simulink model "Demo_TollSystem_cs"  (Simulink 7.6)
settings: Solver=FixedStepDiscrete  SolverMode=SingleTasking  StartTime=0.0  StopTime=13  FixedStep=1/20  RelTol=1e-3
PreLoadFcn:
  | check_NUTS_defined
  | model_closed = 0;
  | assignin('base',['model_closed_' bdroot],false);
InitFcn:
  | PreScanExperimentInitFcn(bdroot)
StopFcn:
  | PreScanExperimentStopFcn(bdroot)
libraries: simulink x9, PreScanUsefulBlocks x6, PreScanSimulinkLibrary x4
(part 2 of 2)

== system Demo_TollSystem_cs/HighwayOverhang_1/RFBeacon_1_Tx_Mux ==
  BeaconType : Inport
  spare_1 : Inport  Port=2
  spare_2 : Inport  Port=3
  spare_3 : Inport  Port=4
  spare_4 : Inport  Port=5
  spare_5 : Inport  Port=6
  spare_6 : Inport  Port=7
  spare_7 : Inport  Port=8
  spare_8 : Inport  Port=9
  spare_9 : Inport  Port=10
  spare_10 : Inport  Port=11
  spare_11 : Inport  Port=12
  spare_12 : Inport  Port=13
  spare_13 : Inport  Port=14
  spare_14 : Inport  Port=15
  spare_15 : Inport  Port=16
  Mux1 : Mux  Inputs=16
  BeaconTx : Outport
  wires:
  BeaconType/1 -> Mux1/1
  spare_11/1 -> Mux1/12
  spare_12/1 -> Mux1/13
  spare_13/1 -> Mux1/14
  spare_14/1 -> Mux1/15
  spare_15/1 -> Mux1/16
  spare_1/1 -> Mux1/2
  spare_2/1 -> Mux1/3
  spare_3/1 -> Mux1/4
  spare_4/1 -> Mux1/5
  spare_5/1 -> Mux1/6
  spare_6/1 -> Mux1/7
  spare_7/1 -> Mux1/8
  spare_8/1 -> Mux1/9
  spare_9/1 -> Mux1/10
  spare_10/1 -> Mux1/11
  Mux1/1 -> BeaconTx/1

== system Demo_TollSystem_cs/HighwayOverhang_1/threshold check ==
  Lat : Inport
  Lon : Inport  Port=2
  Pos Lat : Inport  Port=3
  Pos Lon : Inport  Port=4
  Abs : Abs
  Abs1 : Abs
  Accuracy : Constant  Value=1e-5
  Compare To Zero : simulink/Logic and Bit Operations/Compare To Zero  SystemSampleTime=-1  relop=~=  LogicOutDataTypeMode=uint8  ZeroCross=off
  Compare To Zero1 : simulink/Logic and Bit Operations/Compare To Zero  SystemSampleTime=-1  relop=~=  LogicOutDataTypeMode=uint8  ZeroCross=off
  Logical Operator : Logic  Inputs=3  AllPortsSameDT=off  OutDataTypeStr=boolean
  Logical Operator1 : Logic  Operator=OR  AllPortsSameDT=off  OutDataTypeStr=boolean
  Relational Operator : RelationalOperator  Operator=>  OutDataTypeStr=boolean
  Relational Operator1 : RelationalOperator  Operator=>  OutDataTypeStr=boolean
  Sum : Sum  Inputs=|+-
  Sum1 : Sum  Inputs=|+-
  Out : Outport
  wires:
  Pos Lat/1 -> Sum/2
  Lat/1 -> Sum/1, Compare To Zero/1
  Sum/1 -> Abs/1
  Pos Lon/1 -> Sum1/2
  Lon/1 -> Sum1/1, Compare To Zero1/1
  Sum1/1 -> Abs1/1
  Relational Operator/1 -> Logical Operator1/1
  Logical Operator/1 -> Out/1
  Abs/1 -> Relational Operator/1
  Accuracy/1 -> Relational Operator/2, Relational Operator1/2
  Abs1/1 -> Relational Operator1/1
  Compare To Zero/1 -> Logical Operator/1
  Compare To Zero1/1 -> Logical Operator1/2
  Relational Operator1/1 -> Logical Operator/3
  Logical Operator1/1 -> Logical Operator/2

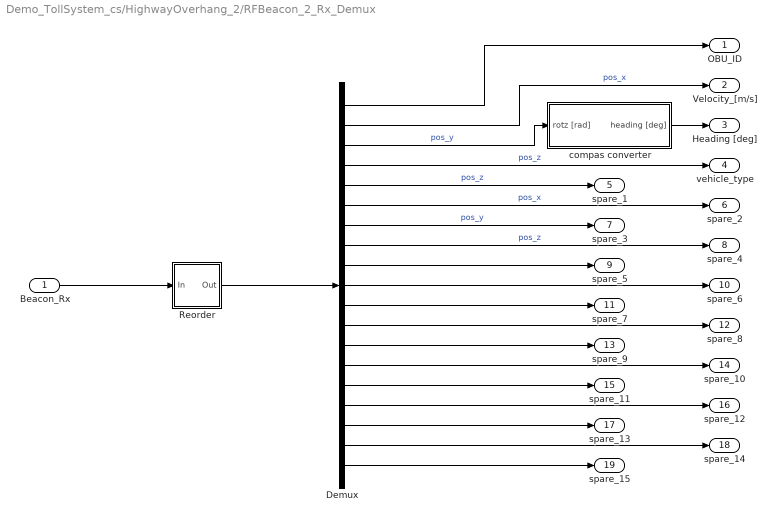
== system Demo_TollSystem_cs/HighwayOverhang_2/RFBeacon_2_Rx_Demux ==
  Beacon_Rx : Inport
  Demux : Demux  Outputs=19
  Reorder : Subsystem  mask(Output reorder block){NrOfOutputs=19, NrOfObjects=5}
      mask prompts: NrOfOutputs "Number Of Outputs [-]"; NrOfObjects "Number Of Objects [-]"
      mask help: Change output order from object based to output type based
      mask init: same as Demo_TollSystem_cs/HighwayOverhang_1/RFBeacon_1_Rx_Demux/Reorder
  compas converter : Subsystem
  OBU_ID : Outport
  Velocity_[m/s] : Outport  Port=2
  Heading [deg] : Outport  Port=3
  vehicle_type : Outport  Port=4
  spare_1 : Outport  Port=5
  spare_2 : Outport  Port=6
  spare_3 : Outport  Port=7
  spare_4 : Outport  Port=8
  spare_5 : Outport  Port=9
  spare_6 : Outport  Port=10
  spare_7 : Outport  Port=11
  spare_8 : Outport  Port=12
  spare_9 : Outport  Port=13
  spare_10 : Outport  Port=14
  spare_11 : Outport  Port=15
  spare_12 : Outport  Port=16
  spare_13 : Outport  Port=17
  spare_14 : Outport  Port=18
  spare_15 : Outport  Port=19
  wires:
  compas converter/1(heading [deg]) -> Heading [deg]/1
  Demux/1 -> OBU_ID/1
  Demux/3 -> compas converter/1(rotz [rad])  "pos_y"
  Demux/2 -> Velocity_[m/s]/1  "pos_x"
  Reorder/1(Out) -> Demux/1
  Demux/5 -> spare_1/1  "pos_z"
  Demux/6 -> spare_2/1  "pos_x"
  Demux/7 -> spare_3/1  "pos_y"
  Demux/8 -> spare_4/1  "pos_z"
  Demux/9 -> spare_5/1
  Demux/10 -> spare_6/1
  Demux/11 -> spare_7/1
  Demux/12 -> spare_8/1
  Demux/13 -> spare_9/1
  Demux/14 -> spare_10/1
  Beacon_Rx/1 -> Reorder/1(In)
  Demux/4 -> vehicle_type/1  "pos_z"
  Demux/15 -> spare_11/1
  Demux/16 -> spare_12/1
  Demux/17 -> spare_13/1
  Demux/18 -> spare_14/1
  Demux/19 -> spare_15/1

== system Demo_TollSystem_cs/HighwayOverhang_2/RFBeacon_2_Tx_Mux ==
  BeaconType : Inport
  spare_1 : Inport  Port=2
  spare_2 : Inport  Port=3
  spare_3 : Inport  Port=4
  spare_4 : Inport  Port=5
  spare_5 : Inport  Port=6
  spare_6 : Inport  Port=7
  spare_7 : Inport  Port=8
  spare_8 : Inport  Port=9
  spare_9 : Inport  Port=10
  spare_10 : Inport  Port=11
  spare_11 : Inport  Port=12
  spare_12 : Inport  Port=13
  spare_13 : Inport  Port=14
  spare_14 : Inport  Port=15
  spare_15 : Inport  Port=16
  Mux1 : Mux  Inputs=16
  BeaconTx : Outport
  wires:
  BeaconType/1 -> Mux1/1
  spare_11/1 -> Mux1/12
  spare_12/1 -> Mux1/13
  spare_13/1 -> Mux1/14
  spare_14/1 -> Mux1/15
  spare_15/1 -> Mux1/16
  spare_1/1 -> Mux1/2
  spare_2/1 -> Mux1/3
  spare_3/1 -> Mux1/4
  spare_4/1 -> Mux1/5
  spare_5/1 -> Mux1/6
  spare_6/1 -> Mux1/7
  spare_7/1 -> Mux1/8
  spare_8/1 -> Mux1/9
  spare_9/1 -> Mux1/10
  spare_10/1 -> Mux1/11
  Mux1/1 -> BeaconTx/1

== system Demo_TollSystem_cs/HighwayOverhang_2/threshold check ==
  Lat : Inport
  Lon : Inport  Port=2
  Pos Lat : Inport  Port=3
  Pos Lon : Inport  Port=4
  Abs : Abs
  Abs1 : Abs
  Accuracy : Constant  Value=1e-5
  Compare To Zero : simulink/Logic and Bit Operations/Compare To Zero  SystemSampleTime=-1  relop=~=  LogicOutDataTypeMode=uint8  ZeroCross=off
  Compare To Zero1 : simulink/Logic and Bit Operations/Compare To Zero  SystemSampleTime=-1  relop=~=  LogicOutDataTypeMode=uint8  ZeroCross=off
  Logical Operator : Logic  Inputs=3  AllPortsSameDT=off  OutDataTypeStr=float('double')
  Logical Operator1 : Logic  Operator=OR  AllPortsSameDT=off  OutDataTypeStr=boolean
  Relational Operator : RelationalOperator  Operator=>  OutDataTypeStr=boolean
  Relational Operator1 : RelationalOperator  Operator=>  OutDataTypeStr=boolean
  Sum : Sum  Inputs=|+-
  Sum1 : Sum  Inputs=|+-
  Out : Outport
  wires:
  Pos Lat/1 -> Sum/2
  Lat/1 -> Sum/1, Compare To Zero/1
  Sum/1 -> Abs/1
  Pos Lon/1 -> Sum1/2
  Lon/1 -> Sum1/1, Compare To Zero1/1
  Sum1/1 -> Abs1/1
  Relational Operator/1 -> Logical Operator1/1
  Logical Operator/1 -> Out/1
  Abs/1 -> Relational Operator/1
  Accuracy/1 -> Relational Operator/2, Relational Operator1/2
  Abs1/1 -> Relational Operator1/1
  Compare To Zero/1 -> Logical Operator/1
  Compare To Zero1/1 -> Logical Operator1/2
  Relational Operator1/1 -> Logical Operator/3
  Logical Operator1/1 -> Logical Operator/2

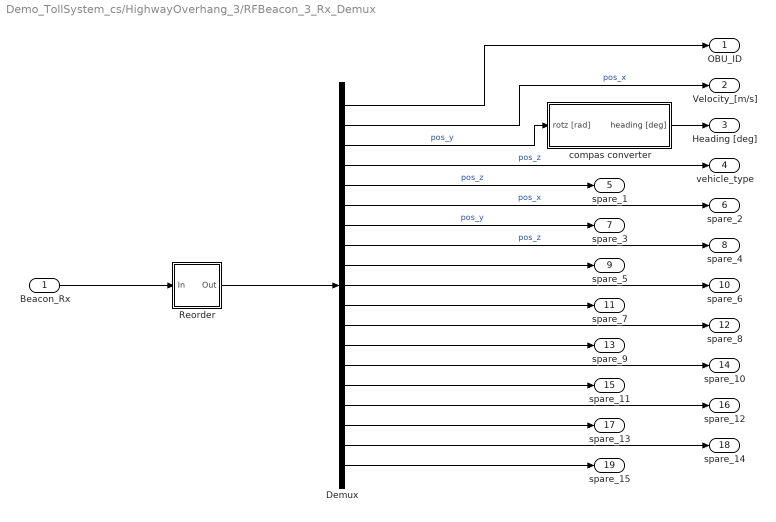
== system Demo_TollSystem_cs/HighwayOverhang_3/RFBeacon_3_Rx_Demux ==
  Beacon_Rx : Inport
  Demux : Demux  Outputs=19
  Reorder : Subsystem  mask(Output reorder block){NrOfOutputs=19, NrOfObjects=5}
      mask prompts: NrOfOutputs "Number Of Outputs [-]"; NrOfObjects "Number Of Objects [-]"
      mask help: Change output order from object based to output type based
      mask init: same as Demo_TollSystem_cs/HighwayOverhang_1/RFBeacon_1_Rx_Demux/Reorder
  compas converter : Subsystem
  OBU_ID : Outport
  Velocity_[m/s] : Outport  Port=2
  Heading [deg] : Outport  Port=3
  vehicle_type : Outport  Port=4
  spare_1 : Outport  Port=5
  spare_2 : Outport  Port=6
  spare_3 : Outport  Port=7
  spare_4 : Outport  Port=8
  spare_5 : Outport  Port=9
  spare_6 : Outport  Port=10
  spare_7 : Outport  Port=11
  spare_8 : Outport  Port=12
  spare_9 : Outport  Port=13
  spare_10 : Outport  Port=14
  spare_11 : Outport  Port=15
  spare_12 : Outport  Port=16
  spare_13 : Outport  Port=17
  spare_14 : Outport  Port=18
  spare_15 : Outport  Port=19
  wires:
  compas converter/1(heading [deg]) -> Heading [deg]/1
  Demux/1 -> OBU_ID/1
  Demux/3 -> compas converter/1(rotz [rad])  "pos_y"
  Demux/2 -> Velocity_[m/s]/1  "pos_x"
  Reorder/1(Out) -> Demux/1
  Demux/5 -> spare_1/1  "pos_z"
  Demux/6 -> spare_2/1  "pos_x"
  Demux/7 -> spare_3/1  "pos_y"
  Demux/8 -> spare_4/1  "pos_z"
  Demux/9 -> spare_5/1
  Demux/10 -> spare_6/1
  Demux/11 -> spare_7/1
  Demux/12 -> spare_8/1
  Demux/13 -> spare_9/1
  Demux/14 -> spare_10/1
  Beacon_Rx/1 -> Reorder/1(In)
  Demux/4 -> vehicle_type/1  "pos_z"
  Demux/15 -> spare_11/1
  Demux/16 -> spare_12/1
  Demux/17 -> spare_13/1
  Demux/18 -> spare_14/1
  Demux/19 -> spare_15/1

== system Demo_TollSystem_cs/HighwayOverhang_3/RFBeacon_3_Tx_Mux ==
  BeaconType : Inport
  spare_1 : Inport  Port=2
  spare_2 : Inport  Port=3
  spare_3 : Inport  Port=4
  spare_4 : Inport  Port=5
  spare_5 : Inport  Port=6
  spare_6 : Inport  Port=7
  spare_7 : Inport  Port=8
  spare_8 : Inport  Port=9
  spare_9 : Inport  Port=10
  spare_10 : Inport  Port=11
  spare_11 : Inport  Port=12
  spare_12 : Inport  Port=13
  spare_13 : Inport  Port=14
  spare_14 : Inport  Port=15
  spare_15 : Inport  Port=16
  Mux1 : Mux  Inputs=16
  BeaconTx : Outport
  wires:
  BeaconType/1 -> Mux1/1
  spare_11/1 -> Mux1/12
  spare_12/1 -> Mux1/13
  spare_13/1 -> Mux1/14
  spare_14/1 -> Mux1/15
  spare_15/1 -> Mux1/16
  spare_1/1 -> Mux1/2
  spare_2/1 -> Mux1/3
  spare_3/1 -> Mux1/4
  spare_4/1 -> Mux1/5
  spare_5/1 -> Mux1/6
  spare_6/1 -> Mux1/7
  spare_7/1 -> Mux1/8
  spare_8/1 -> Mux1/9
  spare_9/1 -> Mux1/10
  spare_10/1 -> Mux1/11
  Mux1/1 -> BeaconTx/1

== system Demo_TollSystem_cs/HighwayOverhang_3/threshold check ==
  Lat : Inport
  Lon : Inport  Port=2
  Pos Lat : Inport  Port=3
  Pos Lon : Inport  Port=4
  Abs : Abs
  Abs1 : Abs
  Accuracy : Constant  Value=1e-5
  Compare To Zero : simulink/Logic and Bit Operations/Compare To Zero  SystemSampleTime=-1  relop=~=  LogicOutDataTypeMode=uint8  ZeroCross=off
  Compare To Zero1 : simulink/Logic and Bit Operations/Compare To Zero  SystemSampleTime=-1  relop=~=  LogicOutDataTypeMode=uint8  ZeroCross=off
  Logical Operator : Logic  Inputs=3  AllPortsSameDT=off  OutDataTypeStr=float('double')
  Logical Operator1 : Logic  Operator=OR  AllPortsSameDT=off  OutDataTypeStr=boolean
  Relational Operator : RelationalOperator  Operator=>  OutDataTypeStr=boolean
  Relational Operator1 : RelationalOperator  Operator=>  OutDataTypeStr=boolean
  Sum : Sum  Inputs=|+-
  Sum1 : Sum  Inputs=|+-
  Out : Outport
  wires:
  Pos Lat/1 -> Sum/2
  Lat/1 -> Sum/1, Compare To Zero/1
  Sum/1 -> Abs/1
  Pos Lon/1 -> Sum1/2
  Lon/1 -> Sum1/1, Compare To Zero1/1
  Sum1/1 -> Abs1/1
  Relational Operator/1 -> Logical Operator1/1
  Logical Operator/1 -> Out/1
  Abs/1 -> Relational Operator/1
  Accuracy/1 -> Relational Operator/2, Relational Operator1/2
  Abs1/1 -> Relational Operator1/1
  Compare To Zero/1 -> Logical Operator/1
  Compare To Zero1/1 -> Logical Operator1/2
  Relational Operator1/1 -> Logical Operator/3
  Logical Operator1/1 -> Logical Operator/2

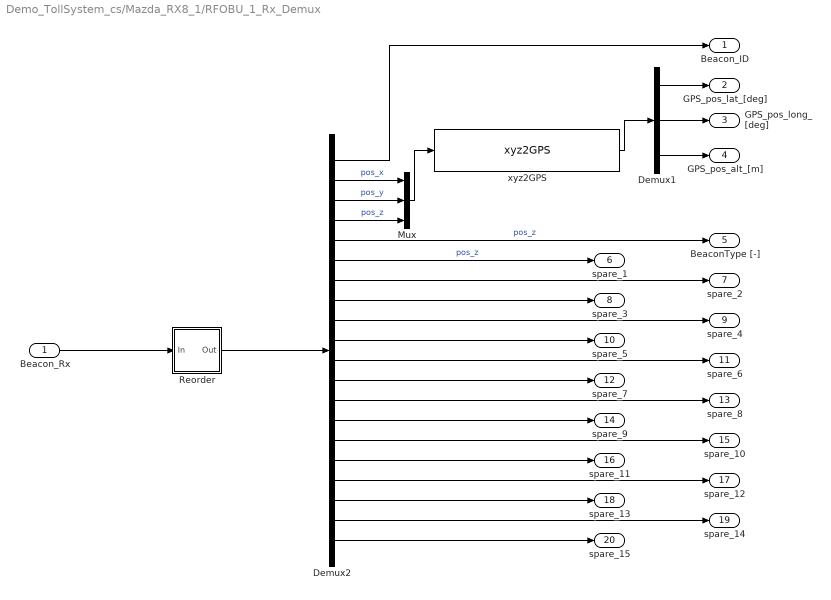
== system Demo_TollSystem_cs/Mazda_RX8_1/RFOBU_1_Rx_Demux ==
  Beacon_Rx : Inport
  Demux1 : Demux  Outputs=3
  Demux2 : Demux  Outputs=20
  Mux : Mux  Inputs=3
  Reorder : Subsystem  mask(Output reorder block){NrOfOutputs=20, NrOfObjects=2}
      mask prompts: NrOfOutputs "Number Of Outputs [-]"; NrOfObjects "Number Of Objects [-]"
      mask help: Change output order from object based to output type based
      mask init: same as Demo_TollSystem_cs/HighwayOverhang_1/RFBeacon_1_Rx_Demux/Reorder
  xyz2GPS : PreScanUsefulBlocks/xyz2GPS  CoordinateCount=2  GPS_base=[52.000000 5.000000 0.000]
  Beacon_ID : Outport
  GPS_pos_lat_[deg] : Outport  Port=2
  GPS_pos_long_[deg] : Outport  Port=3
  GPS_pos_alt_[m] : Outport  Port=4
  BeaconType [-] : Outport  Port=5
  spare_1 : Outport  Port=6
  spare_2 : Outport  Port=7
  spare_3 : Outport  Port=8
  spare_4 : Outport  Port=9
  spare_5 : Outport  Port=10
  spare_6 : Outport  Port=11
  spare_7 : Outport  Port=12
  spare_8 : Outport  Port=13
  spare_9 : Outport  Port=14
  spare_10 : Outport  Port=15
  spare_11 : Outport  Port=16
  spare_12 : Outport  Port=17
  spare_13 : Outport  Port=18
  spare_14 : Outport  Port=19
  spare_15 : Outport  Port=20
  wires:
  Demux2/5 -> BeaconType [-]/1  "pos_z"
  Mux/1 -> xyz2GPS/1
  Demux2/20 -> spare_15/1
  Demux2/19 -> spare_14/1
  Demux2/18 -> spare_13/1
  Demux2/17 -> spare_12/1
  Demux2/16 -> spare_11/1
  Beacon_Rx/1 -> Reorder/1(In)
  Demux2/15 -> spare_10/1
  Demux2/14 -> spare_9/1
  Demux2/13 -> spare_8/1
  Demux2/12 -> spare_7/1
  Demux2/11 -> spare_6/1
  Demux2/10 -> spare_5/1
  Demux2/9 -> spare_4/1
  Demux2/8 -> spare_3/1
  Demux2/7 -> spare_2/1
  Demux2/6 -> spare_1/1  "pos_z"
  Reorder/1(Out) -> Demux2/1
  Demux1/3 -> GPS_pos_alt_[m]/1
  Demux1/2 -> GPS_pos_long_[deg]/1
  Demux1/1 -> GPS_pos_lat_[deg]/1
  xyz2GPS/1 -> Demux1/1
  Demux2/4 -> Mux/3  "pos_z"
  Demux2/3 -> Mux/2  "pos_y"
  Demux2/2 -> Mux/1  "pos_x"
  Demux2/1 -> Beacon_ID/1

== system Demo_TollSystem_cs/Mazda_RX8_1/RFOBU_1_Tx_Mux ==
  Vehicle_Type : Inport
  spare_1 : Inport  Port=2
  spare_2 : Inport  Port=3
  spare_3 : Inport  Port=4
  spare_4 : Inport  Port=5
  spare_5 : Inport  Port=6
  spare_6 : Inport  Port=7
  spare_7 : Inport  Port=8
  spare_8 : Inport  Port=9
  spare_9 : Inport  Port=10
  spare_10 : Inport  Port=11
  spare_11 : Inport  Port=12
  spare_12 : Inport  Port=13
  spare_13 : Inport  Port=14
  spare_14 : Inport  Port=15
  spare_15 : Inport  Port=16
  Mux1 : Mux  Inputs=16
  BeaconTx : Outport
  wires:
  Vehicle_Type/1 -> Mux1/1
  Mux1/1 -> BeaconTx/1
  spare_10/1 -> Mux1/11
  spare_9/1 -> Mux1/10
  spare_8/1 -> Mux1/9
  spare_7/1 -> Mux1/8
  spare_6/1 -> Mux1/7
  spare_5/1 -> Mux1/6
  spare_4/1 -> Mux1/5
  spare_3/1 -> Mux1/4
  spare_2/1 -> Mux1/3
  spare_1/1 -> Mux1/2
  spare_15/1 -> Mux1/16
  spare_14/1 -> Mux1/15
  spare_13/1 -> Mux1/14
  spare_12/1 -> Mux1/13
  spare_11/1 -> Mux1/12

== system Demo_TollSystem_cs/Mazda_RX8_1/S-Memory ==
  note: Memory:
      | - If Set >0 or Rising (switchable)
      |     Out = Signal
      | - Else
      |     Out = Previous Signal
      | - End
  Set : Inport
  Signal : Inport  Port=2
  Detect Rise Positive : simulink/Logic and Bit Operations/Detect Rise Positive  SystemSampleTime=-1  vinit=0
  Manual Switch : simulink/Signal Routing/Manual Switch  SystemSampleTime=-1  sw=1  action=0  varsize=off
  Switch : Switch  Criteria=u2 ~= 0
  Unit Delay : UnitDelay  SampleTime=-1
  Out : Outport
  wires:
  Manual Switch/1 -> Switch/2
  Detect Rise Positive/1 -> Manual Switch/1
  Set/1 -> Manual Switch/2, Detect Rise Positive/1
  Unit Delay/1 -> Switch/3
  Signal/1 -> Switch/1
  Switch/1 -> Unit Delay/1, Out/1

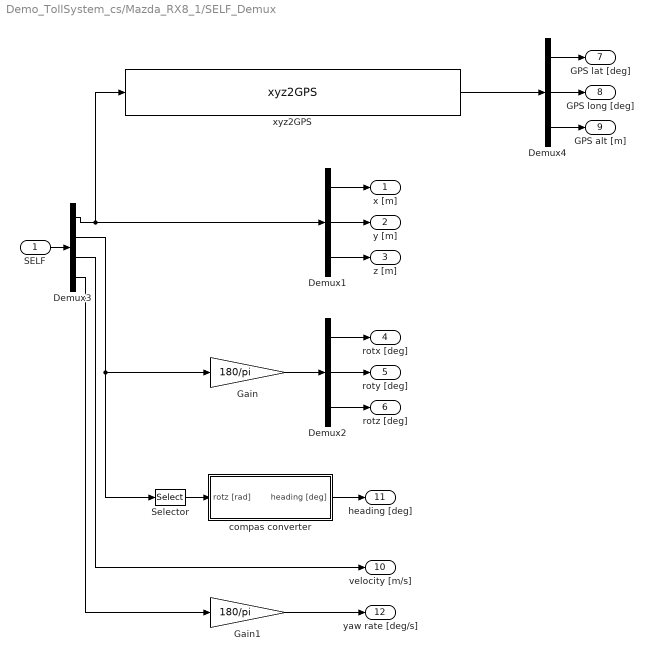
== system Demo_TollSystem_cs/Mazda_RX8_1/SELF_Demux ==
  SELF : Inport
  Demux1 : Demux  Outputs=3
  Demux2 : Demux  Outputs=3
  Demux3 : Demux  Outputs=[3 3 1 1]
  Demux4 : Demux  Outputs=3
  Gain : Gain  Gain=180/pi
  Gain1 : Gain  Gain=180/pi
  Selector : Selector  InputPortWidth=3  IndexOptions=Index vector (dialog)  Indices=[3]  OutputSizes=1
  compas converter : Subsystem
  xyz2GPS : PreScanUsefulBlocks/xyz2GPS  CoordinateCount=1  GPS_base=[52.000000 5.000000 0.000]
  x [m] : Outport
  y [m] : Outport  Port=2
  z [m] : Outport  Port=3
  rotx [deg] : Outport  Port=4
  roty [deg] : Outport  Port=5
  rotz [deg] : Outport  Port=6
  GPS lat [deg] : Outport  Port=7
  GPS long [deg] : Outport  Port=8
  GPS alt [m] : Outport  Port=9
  velocity [m/s] : Outport  Port=10
  heading [deg] : Outport  Port=11
  yaw rate [deg/s] : Outport  Port=12
  wires:
  Demux3/4 -> Gain1/1
  Gain1/1 -> yaw rate [deg/s]/1
  Demux3/3 -> velocity [m/s]/1
  compas converter/1(heading [deg]) -> heading [deg]/1
  xyz2GPS/1 -> Demux4/1
  Demux4/3 -> GPS alt [m]/1
  Demux4/2 -> GPS long [deg]/1
  Demux4/1 -> GPS lat [deg]/1
  Demux3/2 -> Gain/1, Selector/1
  Demux3/1 -> xyz2GPS/1, Demux1/1
  SELF/1 -> Demux3/1
  Demux2/3 -> rotz [deg]/1
  Demux2/2 -> roty [deg]/1
  Demux2/1 -> rotx [deg]/1
  Demux1/3 -> z [m]/1
  Demux1/2 -> y [m]/1
  Demux1/1 -> x [m]/1
  Gain/1 -> Demux2/1
  Selector/1 -> compas converter/1(rotz [rad])

== system Demo_TollSystem_cs/Mazda_RX8_1/Trajectories ==
  PathFollowerSva_1 : Subsystem  Tag=Trajectory  mask(PreScan Source Block: Trajectory){FileName='PathFollowerSva_1.mat', TimeStep=1/20}
      mask prompts: TimeStep "Time Step [s]"
      mask help:
      | The Trajectory block contains the trajectories defined in the PreScan Experiment Editor. The output of the trajectory block is the (vehicle) State.
      |
      | For more information, please click Help.
      mask init:
      | [direc,name]=fileparts(get_param(bdroot, 'FileName'));
      | load([direc,'/Trajectories/',FileName])
      | trajectory=trajectory';
      | 
      | traj.time=trajectory(:,1);%[];
      | traj.signals.values=trajectory(:,2:19);
      | traj.dimensions=18;
      | traj.label='';
      | 
      | SampleTime=traj.time(2)-traj.time(1);
      settings: DeleteFcn=PreScanBlockDeleteFcn;
      mask Help: eval('openHelp(312)')
      mask Display: fprintf(FileName)
  PathFollowerSva_1_Offset : Constant  Tag=TrajectoryOffset  Value="[0  0  0  0  0  0]"
  Traj2State1 : Subsystem  Tag=Traj2State
      settings: DeleteFcn=PreScanBlockDeleteFcn;
      mask Type: PreScan Demux Block:
  State : Outport  Tag=TrajOutport
  wires:
  PathFollowerSva_1/1(trajectory) -> Traj2State1/1(Traj Org)
  PathFollowerSva_1_Offset/1 -> Traj2State1/2(Offset)
  Traj2State1/1(state) -> State/1

== system Demo_TollSystem_cs/STATE_Mazda_RX8_1/Acceleration ==
  Y : Inport
  Assignment : Assignment  IndexMode=Zero-based  SampleTime=TimeStep  IndexOptions=Starting index (dialog)  Indices=PortIndex  OutputSizes=[1 1]
  Data Store Read : DataStoreRead  DataStoreName=SimCoreActuators  SampleTime=TimeStep
  Data Store Write : DataStoreWrite  DataStoreName=SimCoreActuators
  wires:
  Assignment/1 -> Data Store Write/1
  Data Store Read/1 -> Assignment/1
  Y/1 -> Assignment/2

== system Demo_TollSystem_cs/STATE_Mazda_RX8_1/Position ==
  Y : Inport
  Assignment : Assignment  IndexMode=Zero-based  SampleTime=TimeStep  IndexOptions=Starting index (dialog)  Indices=PortIndex  OutputSizes=[1 1]
  Data Store Read : DataStoreRead  DataStoreName=SimCoreActuators  SampleTime=TimeStep
  Data Store Write : DataStoreWrite  DataStoreName=SimCoreActuators
  wires:
  Y/1 -> Assignment/2
  Data Store Read/1 -> Assignment/1
  Assignment/1 -> Data Store Write/1

== system Demo_TollSystem_cs/STATE_Mazda_RX8_1/RPY ==
  Y : Inport
  Assignment : Assignment  IndexMode=Zero-based  SampleTime=TimeStep  IndexOptions=Starting index (dialog)  Indices=PortIndex  OutputSizes=[1 1]
  Data Store Read : DataStoreRead  DataStoreName=SimCoreActuators  SampleTime=TimeStep
  Data Store Write : DataStoreWrite  DataStoreName=SimCoreActuators
  wires:
  Assignment/1 -> Data Store Write/1
  Data Store Read/1 -> Assignment/1
  Y/1 -> Assignment/2

== system Demo_TollSystem_cs/STATE_Mazda_RX8_1/Velocity ==
  Y : Inport
  Assignment : Assignment  IndexMode=Zero-based  SampleTime=TimeStep  IndexOptions=Starting index (dialog)  Indices=PortIndex  OutputSizes=[1 1]
  Data Store Read : DataStoreRead  DataStoreName=SimCoreActuators  SampleTime=TimeStep
  Data Store Write : DataStoreWrite  DataStoreName=SimCoreActuators
  wires:
  Assignment/1 -> Data Store Write/1
  Data Store Read/1 -> Assignment/1
  Y/1 -> Assignment/2

== system Demo_TollSystem_cs/STATE_Mazda_RX8_1/velRPY ==
  Y : Inport
  Assignment : Assignment  IndexMode=Zero-based  SampleTime=TimeStep  IndexOptions=Starting index (dialog)  Indices=PortIndex  OutputSizes=[1 1]
  Data Store Read : DataStoreRead  DataStoreName=SimCoreActuators  SampleTime=TimeStep
  Data Store Write : DataStoreWrite  DataStoreName=SimCoreActuators
  wires:
  Assignment/1 -> Data Store Write/1
  Data Store Read/1 -> Assignment/1
  Y/1 -> Assignment/2

== system Demo_TollSystem_cs/HighwayOverhang_1/RFBeacon_1_Rx_Demux/Reorder ==
  In : Inport
  Selector1 : Selector  InputPortWidth=InputPortWidth  IndexOptions=Index vector (dialog)  Indices=Elements  OutputSizes=1
  Out : Outport
  wires:
  Selector1/1 -> Out/1
  In/1 -> Selector1/1

== system Demo_TollSystem_cs/HighwayOverhang_1/RFBeacon_1_Rx_Demux/compas converter ==
  rotz [rad] : Inport
  cart2compas : Subsystem
  rad2deg : Gain  Gain=180/pi
  heading [deg] : Outport
  wires:
  rad2deg/1 -> cart2compas/1(Angle [deg])
  rotz [rad]/1 -> rad2deg/1
  cart2compas/1(heading [deg]) -> heading [deg]/1

== system Demo_TollSystem_cs/HighwayOverhang_2/RFBeacon_2_Rx_Demux/Reorder ==
  In : Inport
  Selector1 : Selector  InputPortWidth=InputPortWidth  IndexOptions=Index vector (dialog)  Indices=Elements  OutputSizes=1
  Out : Outport
  wires:
  Selector1/1 -> Out/1
  In/1 -> Selector1/1

== system Demo_TollSystem_cs/HighwayOverhang_2/RFBeacon_2_Rx_Demux/compas converter ==
  rotz [rad] : Inport
  cart2compas : Subsystem
  rad2deg : Gain  Gain=180/pi
  heading [deg] : Outport
  wires:
  rad2deg/1 -> cart2compas/1(Angle [deg])
  rotz [rad]/1 -> rad2deg/1
  cart2compas/1(heading [deg]) -> heading [deg]/1

== system Demo_TollSystem_cs/HighwayOverhang_3/RFBeacon_3_Rx_Demux/Reorder ==
  In : Inport
  Selector1 : Selector  InputPortWidth=InputPortWidth  IndexOptions=Index vector (dialog)  Indices=Elements  OutputSizes=1
  Out : Outport
  wires:
  Selector1/1 -> Out/1
  In/1 -> Selector1/1

== system Demo_TollSystem_cs/HighwayOverhang_3/RFBeacon_3_Rx_Demux/compas converter ==
  rotz [rad] : Inport
  cart2compas : Subsystem
  rad2deg : Gain  Gain=180/pi
  heading [deg] : Outport
  wires:
  rad2deg/1 -> cart2compas/1(Angle [deg])
  rotz [rad]/1 -> rad2deg/1
  cart2compas/1(heading [deg]) -> heading [deg]/1

== system Demo_TollSystem_cs/Mazda_RX8_1/RFOBU_1_Rx_Demux/Reorder ==
  In : Inport
  Selector1 : Selector  InputPortWidth=InputPortWidth  IndexOptions=Index vector (dialog)  Indices=Elements  OutputSizes=1
  Out : Outport
  wires:
  In/1 -> Selector1/1
  Selector1/1 -> Out/1

== system Demo_TollSystem_cs/Mazda_RX8_1/SELF_Demux/compas converter ==
  rotz [rad] : Inport
  cart2compas : Subsystem
  rad2deg : Gain  Gain=180/pi
  heading [deg] : Outport
  wires:
  cart2compas/1(heading [deg]) -> heading [deg]/1
  rotz [rad]/1 -> rad2deg/1
  rad2deg/1 -> cart2compas/1(Angle [deg])

== system Demo_TollSystem_cs/Mazda_RX8_1/Trajectories/PathFollowerSva_1 ==
  From Workspace : FromWorkspace  VariableName=trajectory  SampleTime=TimeStep  OutputAfterFinalValue=Holding final value
  From Workspace1 : FromWorkspace  VariableName=trajectory  SampleTime=TimeStep  OutputAfterFinalValue=Setting to zero
  Mux : Mux  Inputs=2
  Selector1 : Selector  InputPortWidth=24  IndexOptions=Index vector (dialog)  Indices=[7:18]  OutputSizes=1
  Selector9 : Selector  InputPortWidth=24  IndexOptions=Index vector (dialog)  Indices=[1:6]  OutputSizes=1
  trajectory : Outport
  wires:
  Selector1/1 -> Mux/2
  Selector9/1 -> Mux/1
  Mux/1 -> trajectory/1
  From Workspace1/1 -> Selector1/1
  From Workspace/1 -> Selector9/1

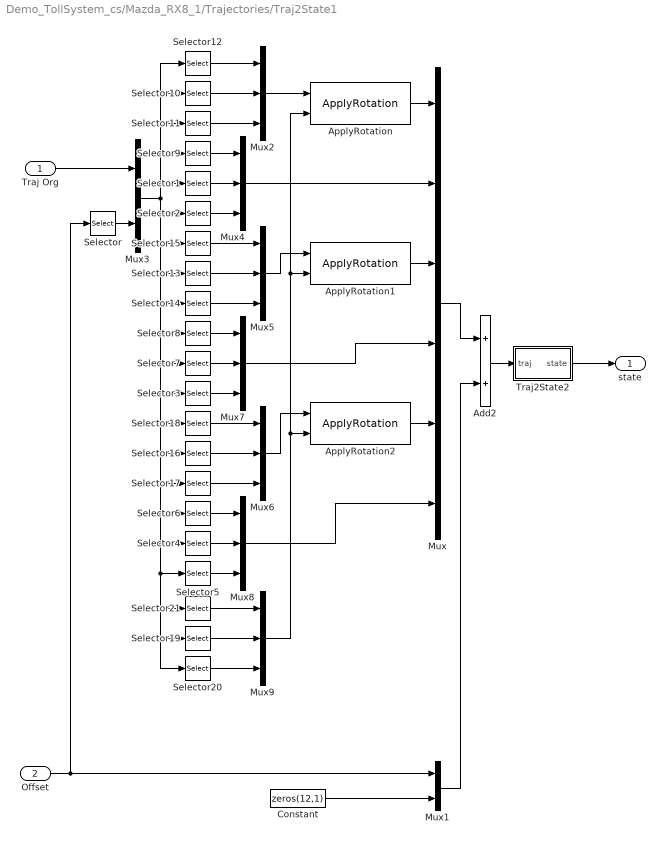
== system Demo_TollSystem_cs/Mazda_RX8_1/Trajectories/Traj2State1 ==
  Traj Org : Inport
  Offset : Inport  Port=2
  Add2 : Sum
  ApplyRotation : PreScanSimulinkLibrary/ApplyRotation  SystemSampleTime=-1
  ApplyRotation1 : PreScanSimulinkLibrary/ApplyRotation  SystemSampleTime=-1
  ApplyRotation2 : PreScanSimulinkLibrary/ApplyRotation  SystemSampleTime=-1
  Constant : Constant  Value=zeros(12,1)
  Mux : Mux  Inputs=6
  Mux1 : Mux  Inputs=2
  Mux{2,4..9} (7 alike) : Mux  Inputs=3
  Mux3 : Mux  Inputs=2
  Selector : Selector  InputPortWidth=6  IndexOptions=Index vector (dialog)  Indices=[4 5 6]  OutputSizes=1
  Selector1 : Selector  InputPortWidth=21  IndexOptions=Index vector (dialog)  Indices=[5]  OutputSizes=1
  Selector10 : Selector  InputPortWidth=21  IndexOptions=Index vector (dialog)  Indices=[2]  OutputSizes=1
  Selector11 : Selector  InputPortWidth=21  IndexOptions=Index vector (dialog)  Indices=[3]  OutputSizes=1
  Selector12 : Selector  InputPortWidth=21  IndexOptions=Index vector (dialog)  Indices=[1]  OutputSizes=1
  Selector13 : Selector  InputPortWidth=21  IndexOptions=Index vector (dialog)  Indices=[8]  OutputSizes=1
  Selector14 : Selector  InputPortWidth=21  IndexOptions=Index vector (dialog)  Indices=[9]  OutputSizes=1
  Selector15 : Selector  InputPortWidth=21  IndexOptions=Index vector (dialog)  Indices=[7]  OutputSizes=1
  Selector16 : Selector  InputPortWidth=21  IndexOptions=Index vector (dialog)  Indices=[14]  OutputSizes=1
  Selector17 : Selector  InputPortWidth=21  IndexOptions=Index vector (dialog)  Indices=[15]  OutputSizes=1
  Selector18 : Selector  InputPortWidth=21  IndexOptions=Index vector (dialog)  Indices=[13]  OutputSizes=1
  Selector19 : Selector  InputPortWidth=21  IndexOptions=Index vector (dialog)  Indices=[20]  OutputSizes=1
  Selector2 : Selector  InputPortWidth=21  IndexOptions=Index vector (dialog)  Indices=[6]  OutputSizes=1
  Selector20 : Selector  InputPortWidth=21  IndexOptions=Index vector (dialog)  Indices=[21]  OutputSizes=1
  Selector21 : Selector  InputPortWidth=21  IndexOptions=Index vector (dialog)  Indices=[19]  OutputSizes=1
  Selector3 : Selector  InputPortWidth=21  IndexOptions=Index vector (dialog)  Indices=[12]  OutputSizes=1
  Selector4 : Selector  InputPortWidth=21  IndexOptions=Index vector (dialog)  Indices=[17]  OutputSizes=1
  Selector5 : Selector  InputPortWidth=21  IndexOptions=Index vector (dialog)  Indices=[18]  OutputSizes=1
  Selector6 : Selector  InputPortWidth=21  IndexOptions=Index vector (dialog)  Indices=[16]  OutputSizes=1
  Selector7 : Selector  InputPortWidth=21  IndexOptions=Index vector (dialog)  Indices=[11]  OutputSizes=1
  Selector8 : Selector  InputPortWidth=21  IndexOptions=Index vector (dialog)  Indices=[10]  OutputSizes=1
  Selector9 : Selector  InputPortWidth=21  IndexOptions=Index vector (dialog)  Indices=[4]  OutputSizes=1
  Traj2State2 : Subsystem
  state : Outport
  wires:
  Mux9/1 -> ApplyRotation2/2, ApplyRotation1/2, ApplyRotation/2
  Selector20/1 -> Mux9/3
  Selector19/1 -> Mux9/2
  Selector21/1 -> Mux9/1
  Selector5/1 -> Mux8/3
  Selector4/1 -> Mux8/2
  Selector6/1 -> Mux8/1
  Mux8/1 -> Mux/6
  Mux6/1 -> ApplyRotation2/1
  Mux7/1 -> Mux/4
  ApplyRotation2/1 -> Mux/5
  Selector3/1 -> Mux7/3
  Selector7/1 -> Mux7/2
  Selector8/1 -> Mux7/1
  Mux4/1 -> Mux/2
  Mux5/1 -> ApplyRotation1/1
  ApplyRotation1/1 -> Mux/3
  Mux2/1 -> ApplyRotation/1
  ApplyRotation/1 -> Mux/1
  Selector2/1 -> Mux4/3
  Selector1/1 -> Mux4/2
  Selector9/1 -> Mux4/1
  Selector17/1 -> Mux6/3
  Selector16/1 -> Mux6/2
  Selector18/1 -> Mux6/1
  Selector14/1 -> Mux5/3
  Selector13/1 -> Mux5/2
  Selector15/1 -> Mux5/1
  Selector11/1 -> Mux2/3
  Selector10/1 -> Mux2/2
  Selector12/1 -> Mux2/1
  Mux3/1 -> Selector8/1, Selector7/1, Selector3/1, Selector18/1, Selector16/1, Selector17/1, Selector6/1, Selector20/1, Selector19/1, Selector21/1, Selector5/1, Selector4/1, Selector14/1, Selector13/1, Selector15/1, Selector2/1, Selector1/1, Selector9/1, Selector12/1, Selector10/1, Selector11/1
  Mux1/1 -> Add2/2
  Constant/1 -> Mux1/2
  Add2/1 -> Traj2State2/1(traj)
  Selector/1 -> Mux3/2
  Traj Org/1 -> Mux3/1
  Offset/1 -> Mux1/1, Selector/1
  Mux/1 -> Add2/1
  Traj2State2/1(state) -> state/1

== system Demo_TollSystem_cs/HighwayOverhang_1/RFBeacon_1_Rx_Demux/compas converter/cart2compas ==
  Angle [deg] : Inport
  Constant : Constant  Value=90
  Constant1 : Constant  Value=360
  Gain : Gain  Gain=1/360
  Gain1 : Gain  Gain=360
  Gain2 : Gain  Gain=-1
  Rounding Function : Rounding
  Sum : Sum  Inputs=|-+
  Sum1 : Sum  Inputs=-+|
  Sum2 : Sum  Inputs=++|
  heading [deg] : Outport
  wires:
  Gain/1 -> Rounding Function/1
  Rounding Function/1 -> Gain1/1
  Gain1/1 -> Sum/1
  Angle [deg]/1 -> Sum1/2
  Sum/1 -> Gain2/1
  Sum1/1 -> Gain/1, Sum/2
  Constant/1 -> Sum1/1
  Gain2/1 -> Sum2/2
  Constant1/1 -> Sum2/1
  Sum2/1 -> heading [deg]/1

== system Demo_TollSystem_cs/HighwayOverhang_2/RFBeacon_2_Rx_Demux/compas converter/cart2compas ==
  Angle [deg] : Inport
  Constant : Constant  Value=90
  Constant1 : Constant  Value=360
  Gain : Gain  Gain=1/360
  Gain1 : Gain  Gain=360
  Gain2 : Gain  Gain=-1
  Rounding Function : Rounding
  Sum : Sum  Inputs=|-+
  Sum1 : Sum  Inputs=-+|
  Sum2 : Sum  Inputs=++|
  heading [deg] : Outport
  wires:
  Gain/1 -> Rounding Function/1
  Rounding Function/1 -> Gain1/1
  Gain1/1 -> Sum/1
  Angle [deg]/1 -> Sum1/2
  Sum/1 -> Gain2/1
  Sum1/1 -> Gain/1, Sum/2
  Constant/1 -> Sum1/1
  Gain2/1 -> Sum2/2
  Constant1/1 -> Sum2/1
  Sum2/1 -> heading [deg]/1

== system Demo_TollSystem_cs/HighwayOverhang_3/RFBeacon_3_Rx_Demux/compas converter/cart2compas ==
  Angle [deg] : Inport
  Constant : Constant  Value=90
  Constant1 : Constant  Value=360
  Gain : Gain  Gain=1/360
  Gain1 : Gain  Gain=360
  Gain2 : Gain  Gain=-1
  Rounding Function : Rounding
  Sum : Sum  Inputs=|-+
  Sum1 : Sum  Inputs=-+|
  Sum2 : Sum  Inputs=++|
  heading [deg] : Outport
  wires:
  Gain/1 -> Rounding Function/1
  Rounding Function/1 -> Gain1/1
  Gain1/1 -> Sum/1
  Angle [deg]/1 -> Sum1/2
  Sum/1 -> Gain2/1
  Sum1/1 -> Gain/1, Sum/2
  Constant/1 -> Sum1/1
  Gain2/1 -> Sum2/2
  Constant1/1 -> Sum2/1
  Sum2/1 -> heading [deg]/1

== system Demo_TollSystem_cs/Mazda_RX8_1/SELF_Demux/compas converter/cart2compas ==
  Angle [deg] : Inport
  Constant : Constant  Value=90
  Constant1 : Constant  Value=360
  Gain : Gain  Gain=1/360
  Gain1 : Gain  Gain=360
  Gain2 : Gain  Gain=-1
  Rounding Function : Rounding
  Sum : Sum  Inputs=|-+
  Sum1 : Sum  Inputs=-+|
  Sum2 : Sum  Inputs=++|
  heading [deg] : Outport
  wires:
  Sum2/1 -> heading [deg]/1
  Constant1/1 -> Sum2/1
  Gain2/1 -> Sum2/2
  Constant/1 -> Sum1/1
  Sum1/1 -> Sum/2, Gain/1
  Sum/1 -> Gain2/1
  Angle [deg]/1 -> Sum1/2
  Gain1/1 -> Sum/1
  Rounding Function/1 -> Gain1/1
  Gain/1 -> Rounding Function/1

== system Demo_TollSystem_cs/Mazda_RX8_1/Trajectories/Traj2State1/Traj2State2 ==
  traj : Inport
  MuxState : Subsystem
  Traj2MuxState_Ext : Subsystem
  state : Outport
  wires:
  Traj2MuxState_Ext/9(Y [rad]) -> MuxState/9(Y [rad])
  Traj2MuxState_Ext/8(P [rad]) -> MuxState/8(P [rad])
  Traj2MuxState_Ext/7(R [rad]) -> MuxState/7(R [rad])
  Traj2MuxState_Ext/6(dz [m/s]) -> MuxState/6(dz [m/s])
  Traj2MuxState_Ext/5(dy [m/s]) -> MuxState/5(dy [m/s])
  Traj2MuxState_Ext/4(dx [m/s]) -> MuxState/4(dx [m/s])
  Traj2MuxState_Ext/3(z [m]) -> MuxState/3(z [m])
  Traj2MuxState_Ext/2(y [m]) -> MuxState/2(y [m])
  Traj2MuxState_Ext/1(x [m]) -> MuxState/1(x [m])
  MuxState/1(state) -> state/1
  traj/1 -> Traj2MuxState_Ext/1(Traj)

== system Demo_TollSystem_cs/Mazda_RX8_1/Trajectories/Traj2State1/Traj2State2/MuxState ==
  x [m] : Inport
  y [m] : Inport  Port=2
  z [m] : Inport  Port=3
  dx [m/s] : Inport  Port=4
  dy [m/s] : Inport  Port=5
  dz [m/s] : Inport  Port=6
  R [rad] : Inport  Port=7
  P [rad] : Inport  Port=8
  Y [rad] : Inport  Port=9
  Mux : Mux  Inputs=9
  state : Outport
  wires:
  z [m]/1 -> Mux/3
  y [m]/1 -> Mux/2
  x [m]/1 -> Mux/1
  Y [rad]/1 -> Mux/9
  P [rad]/1 -> Mux/8
  R [rad]/1 -> Mux/7
  dz [m/s]/1 -> Mux/6
  dy [m/s]/1 -> Mux/5
  dx [m/s]/1 -> Mux/4
  Mux/1 -> state/1

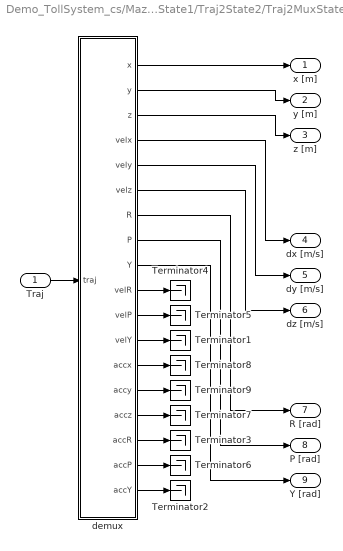
== system Demo_TollSystem_cs/Mazda_RX8_1/Trajectories/Traj2State1/Traj2State2/Traj2MuxState_Ext ==
  Traj : Inport
  Terminator{1..9} (9 alike) : Terminator
  demux : Subsystem
  x [m] : Outport
  y [m] : Outport  Port=2
  z [m] : Outport  Port=3
  dx [m/s] : Outport  Port=4
  dy [m/s] : Outport  Port=5
  dz [m/s] : Outport  Port=6
  R [rad] : Outport  Port=7
  P [rad] : Outport  Port=8
  Y [rad] : Outport  Port=9
  wires:
  demux/9(Y) -> Y [rad]/1
  demux/7(R) -> R [rad]/1
  demux/5(vely) -> dy [m/s]/1
  demux/4(velx) -> dx [m/s]/1
  demux/10(velR) -> Terminator4/1
  demux/11(velP) -> Terminator5/1
  demux/12(velY) -> Terminator1/1
  demux/13(accx) -> Terminator8/1
  demux/14(accy) -> Terminator9/1
  demux/15(accz) -> Terminator7/1
  demux/18(accY) -> Terminator2/1
  demux/16(accR) -> Terminator3/1
  demux/17(accP) -> Terminator6/1
  demux/3(z) -> z [m]/1
  Traj/1 -> demux/1(traj)
  demux/6(velz) -> dz [m/s]/1
  demux/1(x) -> x [m]/1
  demux/2(y) -> y [m]/1
  demux/8(P) -> P [rad]/1

== system Demo_TollSystem_cs/Mazda_RX8_1/Trajectories/Traj2State1/Traj2State2/Traj2MuxState_Ext/demux ==
  traj : Inport
  Demux : Demux  Outputs=18
  x : Outport
  y : Outport  Port=2
  z : Outport  Port=3
  velx : Outport  Port=4
  vely : Outport  Port=5
  velz : Outport  Port=6
  R : Outport  Port=7
  P : Outport  Port=8
  Y : Outport  Port=9
  velR : Outport  Port=10
  velP : Outport  Port=11
  velY : Outport  Port=12
  accx : Outport  Port=13
  accy : Outport  Port=14
  accz : Outport  Port=15
  accR : Outport  Port=16
  accP : Outport  Port=17
  accY : Outport  Port=18
  wires:
  Demux/18 -> accY/1
  Demux/17 -> accP/1
  Demux/16 -> accR/1
  Demux/15 -> accz/1
  Demux/14 -> accy/1
  Demux/13 -> accx/1
  Demux/12 -> velY/1
  Demux/11 -> velP/1
  Demux/10 -> velR/1
  Demux/9 -> velz/1
  Demux/8 -> vely/1
  Demux/7 -> velx/1
  Demux/6 -> Y/1
  Demux/5 -> P/1
  traj/1 -> Demux/1
  Demux/4 -> R/1
  Demux/3 -> z/1
  Demux/2 -> y/1
  Demux/1 -> x/1
